simulink model "CuantNoUnifVoz"  (R2013a)
settings: Solver=ode45  StartTime=0.0  StopTime=1  RelTol=1e-3
values from neighbouring files (symbols this model uses):
  fs = 1/(tout(2)-tout(1))    [CuantNoUniformeVoz.m]    (also in CuantUniformeSeno.m; CuantUniformeVoz.m)
  n = N(i)    [CuantNoUniformeVoz.m]    (also in CuantUniformeSeno.m; CuantUniformeVoz.m)
  xmax = max(entrada)    [CuantNoUniformeVoz.m]
undefined symbols (not defined in the file or in its folder): ln, sgn
settings Model: Creator=Jorge Armando  LastModifiedBy=user
settings DataIOCC: LimitDataPoints=off  SignalLoggingSaveFormat=ModelDataLogs
settings DebuggingCC: MultiTaskDSMMsg=warning  MultiTaskCondExecSysMsg=none  StrictBusMsg=None
settings RTWCC: IncludeERTFirstTime=on
settings GRTTargetCC: CodeReplacementLibrary=None  CPPClassGenCompliant=on

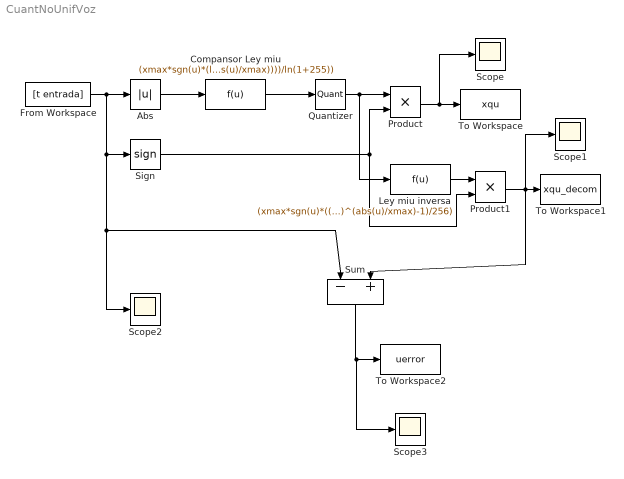
== system CuantNoUnifVoz ==
  Abs : Abs
  Compansor Ley miu : Fcn  Expr=(xmax*sgn(u)*(ln(1+(255*(abs(u)/xmax))))/ln(1+255))
  From Workspace : FromWorkspace  VariableName=[t entrada]  SampleTime=1/fs
  Ley miu inversa : Fcn  Expr=(xmax*sgn(u)*((1+255)^(abs(u)/xmax)-1)/256)
  Product : Product
  Product1 : Product
  Quantizer : Quantizer  QuantizationInterval=1.14*2^(-n)
  Scope{,1..3} (4 alike) : Scope
      Scope2 settings: SaveName=ScopeData2
      Scope3 settings: SaveName=ScopeData3
  Sign : Signum
  Sum : Sum  Inputs=|-+
  To Workspace : ToWorkspace  VariableName=xqu  SampleTime=-1
  To Workspace1 : ToWorkspace  VariableName=xqu_decom  SampleTime=-1
  To Workspace2 : ToWorkspace  VariableName=uerror  SampleTime=-1
  wires:
  From Workspace/1 -> Sign/1, Sum/1, Scope2/1, Abs/1
  Abs/1 -> Compansor Ley miu/1
  Compansor Ley miu/1 -> Quantizer/1
  Quantizer/1 -> Ley miu inversa/1, Product/1
  Sign/1 -> Product1/2, Product/2
  Product/1 -> Scope/1, To Workspace/1
  Ley miu inversa/1 -> Product1/1
  Product1/1 -> Sum/2, Scope1/1, To Workspace1/1
  Sum/1 -> Scope3/1, To Workspace2/1
